simulink model "spi_peripherals"  (R2016b)
settings: Solver=FixedStepDiscrete  StartTime=0.0  StopTime=10.0  FixedStep=1  RelTol=1e-3
undefined symbols (not defined in the file): x2
libraries: mbed_lib x4, mbed_spi_analog_io x3, simulink x2, mbed_spi_several x1, mbed_spi_sensors x1
settings Model: Creator=Stuv  LastModifiedBy=oh
settings DataIOCC: LimitDataPoints=on  SaveFormat=Array
settings OptimizationCC: LifeSpan=1
settings DebuggingCC: SFUnexpectedBacktrackingDiag=warning  SFNoUnconditionalDefaultTransitionDiag=warning  SFExecutionAtInitializationDiag=none
settings HardwareCC: ProdBitPerPointer=32  ProdBitPerSizeT=32  ProdBitPerPtrDiffT=32  ProdLargestAtomicInteger=Long  ProdLargestAtomicFloat=Double  ProdIntDivRoundTo=Undefined  ProdWordSize=32  ProdHWDeviceType=ARM Compatible->ARM Cortex
settings ModelReferenceCC: PropagateSignalLabelsOutOfModel=off
settings RTWCC: SystemTargetFile=mbed.tlc  TemplateMakefile=mbed.tmf  Description=Mbed Target (Embedded Target)  TargetLang=C++
settings CodeAppCC: IgnoreCustomStorageClasses=off
settings STFCustomTargetCC: TargetLibSuffix=.a  GenerateSampleERTMain=on  CombineOutputUpdateFcns=on  ERTCustomFileBanners=on  SupportContinuousTime=off  SupportNonInlinedSFcns=off  RemoveResetFunc=on  MATLABClassNameForMDSCustomization=Simulink.SoftwareTarget.ERTCustomization  GRTInterface=off  SystemTargetFile=mbed.tlc
settings ERTTargetCC: GenerateSampleERTMain=on  ParMdlRefBuildCompliant=off  CompOptLevelCompliant=off  ConcurrentExecutionCompliant=off  ERTFirstTimeCompliant=off  ModelStepFunctionPrototypeControlCompliant=off  CPPClassGenCompliant=off  UseToolchainInfoCompliant=off  ERTCustomFileTemplate=mbed_file_process.tlc  ConvertIfToSwitch=off  SuppressUnreachableDefaultCases=off
settings ConfigComp: CovMetricSettings=dw  CovHtmlReporting=on  CovSaveCumulativeToWorkspaceVar=on  CovSaveSingleToWorkspaceVar=on  CovExternalEMLEnable=off

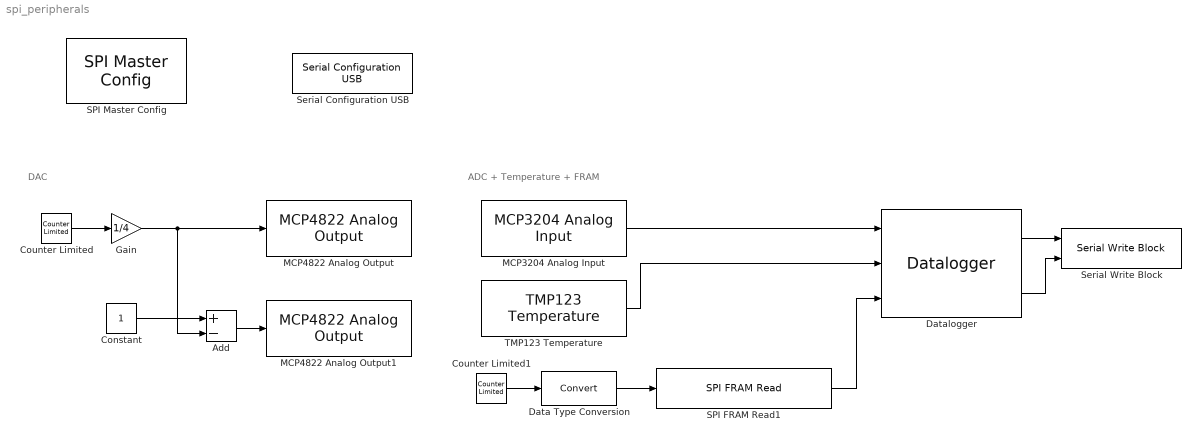
== system spi_peripherals ==
  note: DAC
  note: ADC + Temperature + FRAM
  Add : Sum  Inputs=+-
  Constant : Constant  OutDataTypeStr=single
  Counter Limited : simulink/Sources/Counter Limited  uplimit=4  tsamp=-1
  Counter Limited1 : simulink/Sources/Counter Limited  uplimit=12  tsamp=-1
  Data Type Conversion : DataTypeConversion
  Datalogger : mbed_lib/Utilities/Datalogger  TypeInputPorts={ 'single' 1 'single' 1 'uint8' 1 }  TypeOfInputs={'1*single','1*single','1*uint8'}  BufferSize=40  errEn=off  SampleTime=-1
  Gain : Gain  Gain=1/4  OutDataTypeStr=single
  MCP3204 Analog Input : mbed_spi_analog_io/MCP3204 Analog Input  SpiPort=1  CsPort=A  CsPin=12  Channel=1  Mode=relative  InputType=Single ended  SampleTime=-1
  MCP4822 Analog Output : mbed_spi_analog_io/MCP4822 Analog Output  SpiPort=1  CsPort=A  CsPin=11  Channel=A  Mode=relative  Gain=x2  SampleTime=-1
  MCP4822 Analog Output1 : mbed_spi_analog_io/MCP4822 Analog Output  SpiPort=1  CsPort=A  CsPin=11  Channel=B  Mode=relative  Gain=x2  SampleTime=-1
  SPI FRAM Read1 : mbed_spi_several/SPI FRAM Read  SpiPort=1  CsPort=A  CsPin=0
  SPI Master Config : mbed_lib/Serial/SPI/SPI Master Config  Priority=0  SPIPort=1  Freq=100000  Mode=0  Bits=8  MOSIPortNameShow=A  MOSIPortName=0  MOSIPinNumber=7  MISOPortNameShow=A  MISOPortName=0  MISOPinNumber=6  SCLKPortName=A  Parameter13=0  SCLKPinNumber=5
  Serial Configuration USB : mbed_lib/Serial/UART/Serial Configuration USB  BaudRate=9600
  Serial Write Block : mbed_lib/Serial/UART/Serial Write Block  SerialPort=USB  numData=on  SampleTime=-1
  TMP123 Temperature : mbed_spi_sensors/TMP123 Temperature  SpiPort=1  CsPort=B  CsPin=11  SampleTime=-1
  wires:
  Datalogger/1 -> Serial Write Block/1
  Datalogger/2 -> Serial Write Block/2
  MCP3204 Analog Input/1 -> Datalogger/1
  TMP123 Temperature/1 -> Datalogger/2
  Counter Limited/1 -> Gain/1
  Gain/1 -> MCP4822 Analog Output/1, Add/2
  Constant/1 -> Add/1
  Add/1 -> MCP4822 Analog Output1/1
  SPI FRAM Read1/1 -> Datalogger/3
  Counter Limited1/1 -> Data Type Conversion/1
  Data Type Conversion/1 -> SPI FRAM Read1/1
